simulink model "InvertedPendulumR2020a"  (R2020a)
settings: Solver=VariableStepAuto  StartTime=0.0  StopTime=Inf  RelTol=1e-3
values from neighbouring files (symbols this model uses):
  KD1 = 27.3    [INIT.m]
  KD2 = -0.325    [INIT.m]
  KI1 = 38.3    [INIT.m]
  KI2 = -0.0133    [INIT.m]
  KP1 = 83.2    [INIT.m]
  KP2 = -1.681    [INIT.m]
  LCM = 0.5    [INIT.m]
  Mcart = 0.5    [INIT.m]
  Mpend = 1    [INIT.m]
  Nvar = 0.1    [INIT.m]
  SP = 0.1    [INIT.m]
libraries: vrlib x1
settings Model: Creator=Violet Evergarden  LastModifiedBy=Violet Evergarden

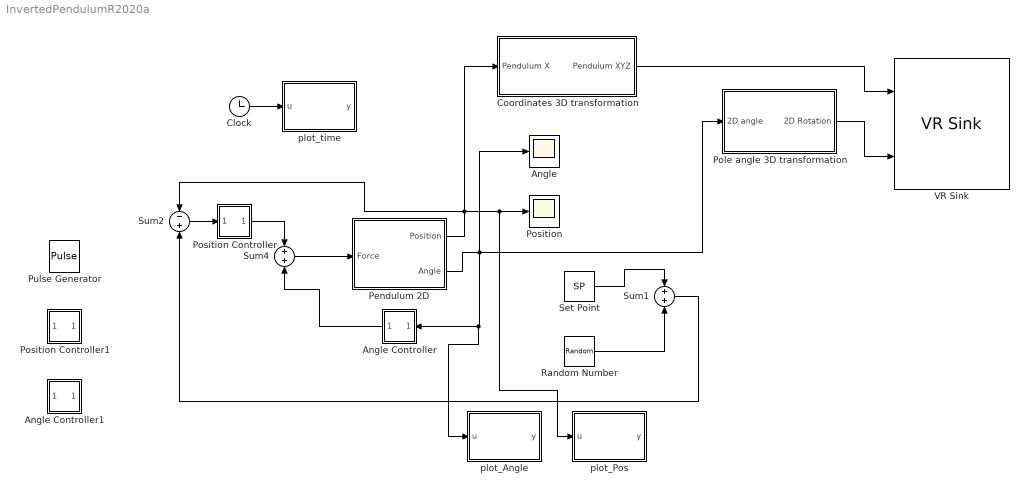
== system InvertedPendulumR2020a ==
  Angle : Scope
  Angle Controller : Subsystem  mask(PID Controller){P=KP1, I=KI1, D=KD1}
      mask prompts: P "Proportional:"; I "Integral:"; D "Derivative:"
      mask help:
      | Enter expressions for proportional, integral, and derivative terms.
      | P+I/s+Ds
      mask Help: This block implements a PID controller where parameters are entered for the Proportional, Integral and Derivative terms. Unmask this block to see how it works. The derivative term is implemented using a true derivative block.
      mask Display: disp('PID')
  Angle Controller1 : Subsystem  mask(PID Controller){P=83.2, I=38.3, D=27.3}
      mask prompts: P "Proportional:"; I "Integral:"; D "Derivative:"
      mask help:
      | Enter expressions for proportional, integral, and derivative terms.
      | P+I/s+Ds
      mask Help: This block implements a PID controller where parameters are entered for the Proportional, Integral and Derivative terms. Unmask this block to see how it works. The derivative term is implemented using a true derivative block.
      mask Display: disp('PID')
  Clock : Clock
  Coordinates 3D transformation : Subsystem
  Pendulum 2D : Subsystem  mask(Inverted pendulum){mc=Mcart, mp=Mpend, l=LCM, g=9.80665}
      mask prompts: mc "Mass of cart (kg):"; mp "Mass of pendulum (kg):"; l "Distance to pendulum center of mass(m):"; g "Acceleration of gravity (m/s^2):"
      mask help: Look under mask to see dynamics
      mask Help: Nonlinear dynamics of inverted pendulum.
      mask Display: plot([-10 10],[0 0],[-2 -2 2 2],[0 1 1 0],[0 -2],[1 5])
  Pole angle 3D transformation : Subsystem
  Position : Scope
  Position Controller : Subsystem  mask(PID Controller){P=KP2, I=KI2, D=KD2}
      mask prompts: P "Proportional:"; I "Integral:"; D "Derivative:"
      mask help:
      | Enter expressions for proportional, integral, and derivative terms.
      | P+I/s+Ds
      mask Help: This block implements a PID controller where parameters are entered for the Proportional, Integral and Derivative terms. Unmask this block to see how it works. The derivative term is implemented using a true derivative block.
      mask Display: disp('PID')
  Position Controller1 : Subsystem  mask(PID Controller){P=-1.681, I=-0.0133, D=-0.325}
      mask prompts: P "Proportional:"; I "Integral:"; D "Derivative:"
      mask help:
      | Enter expressions for proportional, integral, and derivative terms.
      | P+I/s+Ds
      mask Help: This block implements a PID controller where parameters are entered for the Proportional, Integral and Derivative terms. Unmask this block to see how it works. The derivative term is implemented using a true derivative block.
      mask Display: disp('PID')
  Pulse Generator : DiscretePulseGenerator  PulseType=Time based  Amplitude=100  Period=10  PulseWidth=0.01
  Random Number : RandomNumber  Variance=Nvar  Seed=0.1  SampleTime=3
  Set Point : Constant  Value=SP
  Sum1 : Sum  InputSameDT=on  SaturateOnIntegerOverflow=on  OutDataTypeStr=Inherit: Same as first input
  Sum2 : Sum  Inputs=-+  InputSameDT=on  SaturateOnIntegerOverflow=on  OutDataTypeStr=Inherit: Same as first input
  Sum4 : Sum  InputSameDT=on  SaturateOnIntegerOverflow=on  OutDataTypeStr=Inherit: Same as first input
  VR Sink : vrlib/VR Sink  InstantiateOnLoad=on  SampleTime=0.2  ViewEnable=on  RemoteChange=off  RemoteView=off  FieldsWritten=Pendulum.translation.3.1.1.double#Pole1.rotation.4.1.1.double  WorldFileName=pendulum_vr.wrl  WorldDescription=Inverted Pendulum  AutoView=on  VideoDimensions=[]  AllowVariableSize=off  FigureProperties="{'Position', 'Name', 'Viewpoint', 'CameraBound', 'CameraDirection', 'CameraPosition', 'CameraUpVector', 'ZoomFactor', 'Antialiasing', 'Headlight', 'Lighting', 'NavPanel', 'Sound', 'StatusBar', 'Stereo3D', 'Stereo3DCameraOffset', 'Stereo3DHIT', 'ToolBar', 'Textures', 'Transparency', 'Triad', 'Wireframe', 'NavZones', 'NavMode', 'NavSpeed', 'CaptureFileFormat', 'CaptureFileName', 'Record2DCompressMethod', 'Record2DCompressQuality', 'Record2D', 'Record2DFileName', 'Record2DFPS'; [2.0000000000000000e+00   9.2000000000000000e+01   5.7600000000000000e+02   3.5000000000000000e+02], 'Inverted Pendulum', 'Front view', 'on', [0.0000000000000000e+00   0.0000000000000000e+00  -1.0000000000000000e+00], [0.0000000000000000e+00   0.0000000000000000e+00   0.0000000000000000e+00], [0.0000000000000000e+00   1.0000000000000000e+00   0.0000000000000000e+00], [1.0000000000000000e+00], 'on', 'on', 'on', 'halfbar', 'on', 'on', 'off', [1.0000000149011612e-01], [0.0000000000000000e+00], 'on', 'on', 'on', 'none', 'off', 'off', 'examine', 'normal', 'tif', '%f_anim_%n.tif', 'auto', [7.5000000000000000e+01], 'off', '%f_anim_%n.avi', 'auto'}"
  plot_Angle : MATLAB Function  TreatAsAtomicUnit=on
  plot_Pos : MATLAB Function  TreatAsAtomicUnit=on
  plot_time : MATLAB Function  TreatAsAtomicUnit=on
  wires:
  Position Controller/1(Out_1) -> Sum4/1
  Sum2/1 -> Position Controller/1(In_1)
  Pendulum 2D/1(Position) -> Sum2/1, Coordinates 3D transformation/1(Pendulum X), plot_Pos/1(u), Position/1
  Pendulum 2D/2(Angle) -> plot_Angle/1(u), Angle Controller/1(In_1), Pole angle 3D transformation/1(2D angle), Angle/1
  Angle Controller/1(Out_1) -> Sum4/2
  Sum1/1 -> Sum2/2
  Set Point/1 -> Sum1/1
  Sum4/1 -> Pendulum 2D/1(Force)
  Random Number/1 -> Sum1/2
  Coordinates 3D transformation/1(Pendulum XYZ) -> VR Sink/1
  Pole angle 3D transformation/1(2D Rotation) -> VR Sink/2
  Clock/1 -> plot_time/1(u)

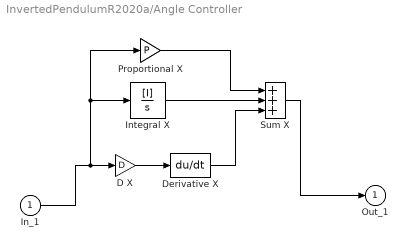
== system InvertedPendulumR2020a/Angle Controller ==
  In_1 : Inport
  D X : Gain  Gain=D  SaturateOnIntegerOverflow=on  OutDataTypeStr=Inherit: Same as input  ParamDataTypeStr=Inherit: Same as input
  Derivative X : Derivative
  Integral X : TransferFcn  Numerator=[I]  Denominator=[1 0]
  Proportional X : Gain  Gain=P  SaturateOnIntegerOverflow=on  OutDataTypeStr=Inherit: Same as input  ParamDataTypeStr=Inherit: Same as input
  Sum X : Sum  Inputs=+++  InputSameDT=on  SaturateOnIntegerOverflow=on  OutDataTypeStr=Inherit: Same as first input
  Out_1 : Outport  InitialOutput=0  VectorParamsAs1DForOutWhenUnconnected=off
  wires:
  D X/1 -> Derivative X/1
  Derivative X/1 -> Sum X/3
  Integral X/1 -> Sum X/2
  Proportional X/1 -> Sum X/1
  In_1/1 -> D X/1, Integral X/1, Proportional X/1
  Sum X/1 -> Out_1/1

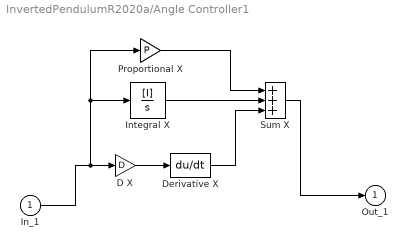
== system InvertedPendulumR2020a/Angle Controller1 ==
  In_1 : Inport
  D X : Gain  Gain=D  SaturateOnIntegerOverflow=on  OutDataTypeStr=Inherit: Same as input  ParamDataTypeStr=Inherit: Same as input
  Derivative X : Derivative
  Integral X : TransferFcn  Numerator=[I]  Denominator=[1 0]
  Proportional X : Gain  Gain=P  SaturateOnIntegerOverflow=on  OutDataTypeStr=Inherit: Same as input  ParamDataTypeStr=Inherit: Same as input
  Sum X : Sum  Inputs=+++  InputSameDT=on  SaturateOnIntegerOverflow=on  OutDataTypeStr=Inherit: Same as first input
  Out_1 : Outport  InitialOutput=0  VectorParamsAs1DForOutWhenUnconnected=off
  wires:
  Sum X/1 -> Out_1/1
  In_1/1 -> Proportional X/1, Integral X/1, D X/1
  Proportional X/1 -> Sum X/1
  Integral X/1 -> Sum X/2
  Derivative X/1 -> Sum X/3
  D X/1 -> Derivative X/1

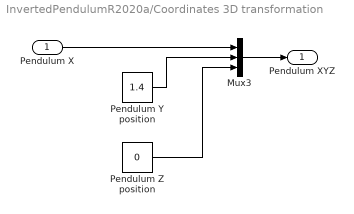
== system InvertedPendulumR2020a/Coordinates 3D transformation ==
  Pendulum X : Inport
  Mux3 : Mux  Inputs=3
  Pendulum Y position : Constant  Value=1.4
  Pendulum Z position : Constant  Value=0
  Pendulum XYZ : Outport  VectorParamsAs1DForOutWhenUnconnected=off
  wires:
  Pendulum Y position/1 -> Mux3/2
  Mux3/1 -> Pendulum XYZ/1
  Pendulum X/1 -> Mux3/1
  Pendulum Z position/1 -> Mux3/3

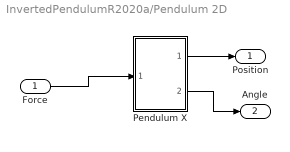
== system InvertedPendulumR2020a/Pendulum 2D ==
  Force : Inport
  Pendulum X : Subsystem  mask(Inverted pendulum){mc=mc, mp=mp, l=l, g=g}
      mask prompts: mc "Mass of cart (kg):"; mp "Mass of pendulum (kg):"; l "Distance to pendulum center of mass(m):"; g "Acceleration of gravity (m/s^2):"
      mask help: Look under mask to see dynamics
      mask Help: Nonlinear dynamics of inverted pendulum.
  Position : Outport  VectorParamsAs1DForOutWhenUnconnected=off
  Angle : Outport  Port=2  VectorParamsAs1DForOutWhenUnconnected=off
  wires:
  Force/1 -> Pendulum X/1(Force)
  Pendulum X/1(Position) -> Position/1
  Pendulum X/2(Angle) -> Angle/1

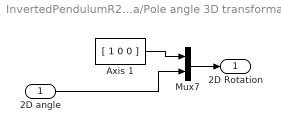
== system InvertedPendulumR2020a/Pole angle 3D transformation ==
  2D angle : Inport
  Axis 1 : Constant  Value=[ 1 0 0 ]
  Mux7 : Mux  Inputs=2
  2D Rotation : Outport  VectorParamsAs1DForOutWhenUnconnected=off
  wires:
  Axis 1/1 -> Mux7/1
  Mux7/1 -> 2D Rotation/1
  2D angle/1 -> Mux7/2

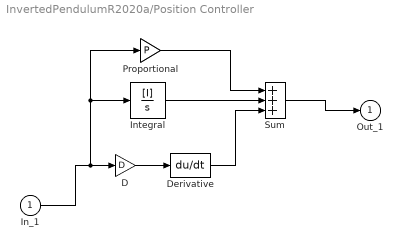
== system InvertedPendulumR2020a/Position Controller ==
  In_1 : Inport
  D : Gain  Gain=D  SaturateOnIntegerOverflow=on  OutDataTypeStr=Inherit: Same as input  ParamDataTypeStr=Inherit: Same as input
  Derivative : Derivative
  Integral : TransferFcn  Numerator=[I]  Denominator=[1 0]
  Proportional : Gain  Gain=P  SaturateOnIntegerOverflow=on  OutDataTypeStr=Inherit: Same as input  ParamDataTypeStr=Inherit: Same as input
  Sum : Sum  Inputs=+++  InputSameDT=on  SaturateOnIntegerOverflow=on  OutDataTypeStr=Inherit: Same as first input
  Out_1 : Outport  InitialOutput=0  VectorParamsAs1DForOutWhenUnconnected=off
  wires:
  Sum/1 -> Out_1/1
  In_1/1 -> Proportional/1, Integral/1, D/1
  Proportional/1 -> Sum/1
  Integral/1 -> Sum/2
  Derivative/1 -> Sum/3
  D/1 -> Derivative/1

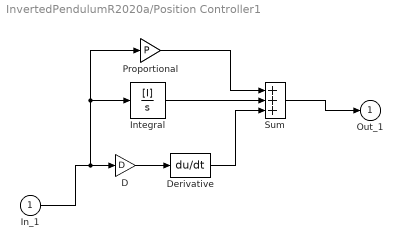
== system InvertedPendulumR2020a/Position Controller1 ==
  In_1 : Inport
  D : Gain  Gain=D  SaturateOnIntegerOverflow=on  OutDataTypeStr=Inherit: Same as input  ParamDataTypeStr=Inherit: Same as input
  Derivative : Derivative
  Integral : TransferFcn  Numerator=[I]  Denominator=[1 0]
  Proportional : Gain  Gain=P  SaturateOnIntegerOverflow=on  OutDataTypeStr=Inherit: Same as input  ParamDataTypeStr=Inherit: Same as input
  Sum : Sum  Inputs=+++  InputSameDT=on  SaturateOnIntegerOverflow=on  OutDataTypeStr=Inherit: Same as first input
  Out_1 : Outport  InitialOutput=0  VectorParamsAs1DForOutWhenUnconnected=off
  wires:
  D/1 -> Derivative/1
  Derivative/1 -> Sum/3
  Integral/1 -> Sum/2
  Proportional/1 -> Sum/1
  In_1/1 -> D/1, Integral/1, Proportional/1
  Sum/1 -> Out_1/1

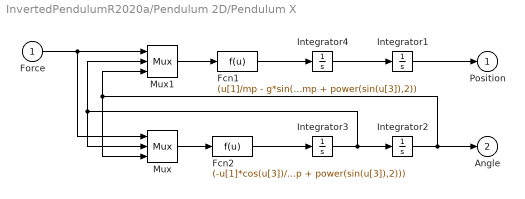
== system InvertedPendulumR2020a/Pendulum 2D/Pendulum X ==
  Force : Inport
  Fcn1 : Fcn  Expr=(u[1]/mp - g*sin(u[3])*cos(u[3]) + l*power(u[2],2)*sin(u[3]))/(mc/mp + power(sin(u[3]),2))
  Fcn2 : Fcn  Expr=(-u[1]*cos(u[3])/mp + (mc+mp)*g*sin(u[3])/mp - l*power(u[2],2)*sin(u[3])*cos(u[3]))/(l*(mc/mp + power(sin(u[3]),2)))
  Integrator1 : Integrator  UpperSaturationLimit=Inf  LowerSaturationLimit=-Inf  ZeroCross=off
  Integrator2 : Integrator  LimitOutput=on  UpperSaturationLimit=pi/2  LowerSaturationLimit=-pi/2  ZeroCross=off
  Integrator3 : Integrator  UpperSaturationLimit=Inf  LowerSaturationLimit=-Inf  ZeroCross=off
  Integrator4 : Integrator  UpperSaturationLimit=Inf  LowerSaturationLimit=-Inf  ZeroCross=off
  Mux : Mux  Inputs=3
  Mux1 : Mux  Inputs=3
  Position : Outport  InitialOutput=0  VectorParamsAs1DForOutWhenUnconnected=off
  Angle : Outport  Port=2  InitialOutput=0  VectorParamsAs1DForOutWhenUnconnected=off
  wires:
  Integrator2/1 -> Mux/3, Mux1/3, Angle/1
  Integrator3/1 -> Mux/2, Mux1/2, Integrator2/1
  Force/1 -> Mux/1, Mux1/1
  Integrator4/1 -> Integrator1/1
  Fcn1/1 -> Integrator4/1
  Mux1/1 -> Fcn1/1
  Mux/1 -> Fcn2/1
  Fcn2/1 -> Integrator3/1
  Integrator1/1 -> Position/1

== matlab function InvertedPendulumR2020a/plot_time ==
  data: u input; y output
function y = run_time(u)

y = u;

== matlab function InvertedPendulumR2020a/plot_Pos ==
  data: u input; y output
function y = plot_Pos(u)

y = u;

== matlab function InvertedPendulumR2020a/plot_Angle ==
  data: u input; y output
function y = plot_Angle(u)

y = u;
